simulink model "ZieglerTu4_102"  (Simulink 5.0)
settings: Solver=ode4  StartTime=0.0  StopTime=15  FixedStep=0.001  RelTol=1e-3
libraries: simulink_extras x1
settings Model: LastModifiedBy=ThinkPad  ExtModeTrigMode=oneshot  ExtModeArmWhenConnect=off  LimitDataPoints=off  BooleanDataType=off

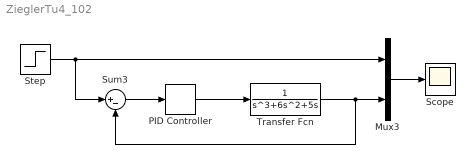
== system ZieglerTu4_102 ==
  Mux3 : Mux  Inputs=2
  PID Controller : simulink_extras/Additional Linear/PID Controller  P=30  I=0  D=0
  "Scope " : Scope
      settings: YMin=-3.5  YMax=1  SaveName=ZieglermTu4_102  DataFormat=Array  MaxDataPoints=500000
  Step : Step  Time=0  SampleTime=0
  Sum3 : Sum  Inputs=|+-  SaturateOnIntegerOverflow=on
  "Transfer Fcn " : TransferFcn  Denominator=[1,6,5 0]
  wires:
  Step/1 -> Sum3/1, Mux3/1
  Mux3/1 -> "Scope "/1
  "Transfer Fcn "/1 -> Sum3/2, Mux3/2
  PID Controller/1 -> "Transfer Fcn "/1
  Sum3/1 -> PID Controller/1
